simulink model "DC_Motor_Model"  (R2020b)
settings: Solver=VariableStepAuto  StartTime=0.0  StopTime=50  RelTol=1e-3
values from neighbouring files (symbols this model uses):
  B = 0.004    [Robot_Parameters.m]
  J = 0.0363    [Robot_Parameters.m]
  Ke = 0.03    [Robot_Parameters.m]
  Kt = 0.001    [Robot_Parameters.m]
  L = 0.01    [Robot_Parameters.m]
  N = 30    [Robot_Parameters.m]
  R = 0.7    [Robot_Parameters.m]
settings Model: OrderedModelArguments=off  Creator=dell  LastModifiedBy=dell

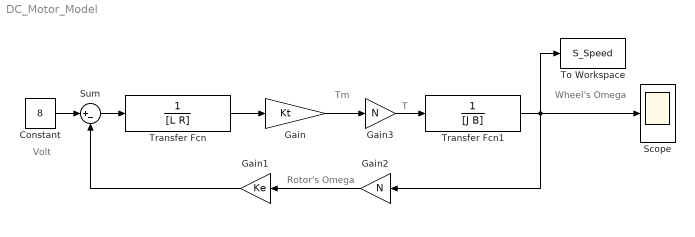
== system DC_Motor_Model ==
  note: Rotor's Omega
  note: Wheel's Omega
  note: T
  note: Tm
  note: Volt
  Constant : Constant  Value=8
  Gain : Gain  Gain=Kt
  Gain1 : Gain  Gain=Ke
  Gain2 : Gain  Gain=N
  Gain3 : Gain  Gain=N
  Scope : Scope
  Sum : Sum  Inputs=|+-
  To Workspace : ToWorkspace  VariableName=S_Speed  SaveFormat=Timeseries  SampleTime=1
  Transfer Fcn : TransferFcn  Denominator=[L R]
  Transfer Fcn1 : TransferFcn  Denominator=[J B]
  wires:
  Sum/1 -> Transfer Fcn/1
  Transfer Fcn/1 -> Gain/1
  Transfer Fcn1/1 -> Gain2/1, Scope/1, To Workspace/1
  Gain1/1 -> Sum/2
  Constant/1 -> Sum/1
  Gain2/1 -> Gain1/1
  Gain/1 -> Gain3/1
  Gain3/1 -> Transfer Fcn1/1
